simulink model "pfb_fir_generic_test_sim4"  (R2012b)
settings: Solver=VariableStepDiscrete  StartTime=0.0  StopTime=10.0  RelTol=1e-3
model workspace (MAT data in the model file):
  synci = [0 1 2 3 4 5 6 7 8 9 10 11 ... (589826 elements, 294913x2)]
  din0 = [0 1 2 3 4 5 6 7 8 9 10 11 ... (73730 elements, 36865x2)]
  din1 = [0 1 2 3 4 5 6 7 8 9 10 11 ... (73730 elements, 36865x2)]
  din2 = [0 1 2 3 4 5 6 7 8 9 10 11 ... (73730 elements, 36865x2)]
  din3 = [0 1 2 3 4 5 6 7 8 9 10 11 ... (73730 elements, 36865x2)]
  din4 = [0 1 2 3 4 5 6 7 8 9 10 11 ... (73730 elements, 36865x2)]
  din5 = [0 1 2 3 4 5 6 7 8 9 10 11 ... (73730 elements, 36865x2)]
  din6 = [0 1 2 3 4 5 6 7 8 9 10 11 ... (73730 elements, 36865x2)]
  din7 = [0 1 2 3 4 5 6 7 8 9 10 11 ... (73730 elements, 36865x2)]
libraries: xbsIndex_r4 x5323, casper_library_delays x1
(part 16 of 23)

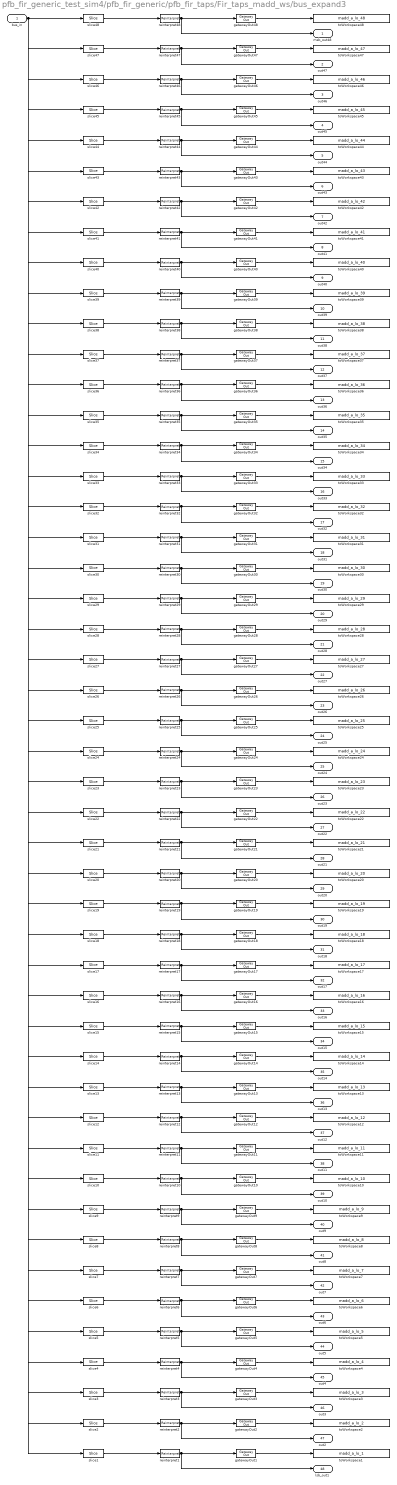
== system pfb_fir_generic_test_sim4/pfb_fir_generic/pfb_fir_taps/Fir_taps_madd_ws/bus_expand3 ==
  bus_in : Inport
  gatewayOut{1..48} (48 alike) : xbsIndex_r4/Gateway Out  inherit_from_input=off  hdl_port=off  timing_constraint=None  locs_specified=off  LOCs={}  UseAsDAC=off  DACChannel='1'  block_type=gatewayout
  reinterpret{1..48} (48 alike) : xbsIndex_r4/Reinterpret  force_arith_type=on  arith_type="Signed  (2's comp)"  force_bin_pt=on  bin_pt=9  block_type=reinterpret
  slice1 : xbsIndex_r4/Slice  nbits=10  boolean_output=off  mode=Upper Bit Location + Width  bit1=-470  base1=MSB of Input  bit0=0  base0=LSB of Input  dbl_ovrd=off  block_type=slice
  slice10 : xbsIndex_r4/Slice  nbits=10  boolean_output=off  mode=Upper Bit Location + Width  bit1=-380  base1=MSB of Input  bit0=0  base0=LSB of Input  dbl_ovrd=off  block_type=slice
  slice11 : xbsIndex_r4/Slice  nbits=10  boolean_output=off  mode=Upper Bit Location + Width  bit1=-370  base1=MSB of Input  bit0=0  base0=LSB of Input  dbl_ovrd=off  block_type=slice
  slice12 : xbsIndex_r4/Slice  nbits=10  boolean_output=off  mode=Upper Bit Location + Width  bit1=-360  base1=MSB of Input  bit0=0  base0=LSB of Input  dbl_ovrd=off  block_type=slice
  slice13 : xbsIndex_r4/Slice  nbits=10  boolean_output=off  mode=Upper Bit Location + Width  bit1=-350  base1=MSB of Input  bit0=0  base0=LSB of Input  dbl_ovrd=off  block_type=slice
  slice14 : xbsIndex_r4/Slice  nbits=10  boolean_output=off  mode=Upper Bit Location + Width  bit1=-340  base1=MSB of Input  bit0=0  base0=LSB of Input  dbl_ovrd=off  block_type=slice
  slice15 : xbsIndex_r4/Slice  nbits=10  boolean_output=off  mode=Upper Bit Location + Width  bit1=-330  base1=MSB of Input  bit0=0  base0=LSB of Input  dbl_ovrd=off  block_type=slice
  slice16 : xbsIndex_r4/Slice  nbits=10  boolean_output=off  mode=Upper Bit Location + Width  bit1=-320  base1=MSB of Input  bit0=0  base0=LSB of Input  dbl_ovrd=off  block_type=slice
  slice17 : xbsIndex_r4/Slice  nbits=10  boolean_output=off  mode=Upper Bit Location + Width  bit1=-310  base1=MSB of Input  bit0=0  base0=LSB of Input  dbl_ovrd=off  block_type=slice
  slice18 : xbsIndex_r4/Slice  nbits=10  boolean_output=off  mode=Upper Bit Location + Width  bit1=-300  base1=MSB of Input  bit0=0  base0=LSB of Input  dbl_ovrd=off  block_type=slice
  slice19 : xbsIndex_r4/Slice  nbits=10  boolean_output=off  mode=Upper Bit Location + Width  bit1=-290  base1=MSB of Input  bit0=0  base0=LSB of Input  dbl_ovrd=off  block_type=slice
  slice2 : xbsIndex_r4/Slice  nbits=10  boolean_output=off  mode=Upper Bit Location + Width  bit1=-460  base1=MSB of Input  bit0=0  base0=LSB of Input  dbl_ovrd=off  block_type=slice
  slice20 : xbsIndex_r4/Slice  nbits=10  boolean_output=off  mode=Upper Bit Location + Width  bit1=-280  base1=MSB of Input  bit0=0  base0=LSB of Input  dbl_ovrd=off  block_type=slice
  slice21 : xbsIndex_r4/Slice  nbits=10  boolean_output=off  mode=Upper Bit Location + Width  bit1=-270  base1=MSB of Input  bit0=0  base0=LSB of Input  dbl_ovrd=off  block_type=slice
  slice22 : xbsIndex_r4/Slice  nbits=10  boolean_output=off  mode=Upper Bit Location + Width  bit1=-260  base1=MSB of Input  bit0=0  base0=LSB of Input  dbl_ovrd=off  block_type=slice
  slice23 : xbsIndex_r4/Slice  nbits=10  boolean_output=off  mode=Upper Bit Location + Width  bit1=-250  base1=MSB of Input  bit0=0  base0=LSB of Input  dbl_ovrd=off  block_type=slice
  slice24 : xbsIndex_r4/Slice  nbits=10  boolean_output=off  mode=Upper Bit Location + Width  bit1=-240  base1=MSB of Input  bit0=0  base0=LSB of Input  dbl_ovrd=off  block_type=slice
  slice25 : xbsIndex_r4/Slice  nbits=10  boolean_output=off  mode=Upper Bit Location + Width  bit1=-230  base1=MSB of Input  bit0=0  base0=LSB of Input  dbl_ovrd=off  block_type=slice
  slice26 : xbsIndex_r4/Slice  nbits=10  boolean_output=off  mode=Upper Bit Location + Width  bit1=-220  base1=MSB of Input  bit0=0  base0=LSB of Input  dbl_ovrd=off  block_type=slice
  slice27 : xbsIndex_r4/Slice  nbits=10  boolean_output=off  mode=Upper Bit Location + Width  bit1=-210  base1=MSB of Input  bit0=0  base0=LSB of Input  dbl_ovrd=off  block_type=slice
  slice28 : xbsIndex_r4/Slice  nbits=10  boolean_output=off  mode=Upper Bit Location + Width  bit1=-200  base1=MSB of Input  bit0=0  base0=LSB of Input  dbl_ovrd=off  block_type=slice
  slice29 : xbsIndex_r4/Slice  nbits=10  boolean_output=off  mode=Upper Bit Location + Width  bit1=-190  base1=MSB of Input  bit0=0  base0=LSB of Input  dbl_ovrd=off  block_type=slice
  slice3 : xbsIndex_r4/Slice  nbits=10  boolean_output=off  mode=Upper Bit Location + Width  bit1=-450  base1=MSB of Input  bit0=0  base0=LSB of Input  dbl_ovrd=off  block_type=slice
  slice30 : xbsIndex_r4/Slice  nbits=10  boolean_output=off  mode=Upper Bit Location + Width  bit1=-180  base1=MSB of Input  bit0=0  base0=LSB of Input  dbl_ovrd=off  block_type=slice
  slice31 : xbsIndex_r4/Slice  nbits=10  boolean_output=off  mode=Upper Bit Location + Width  bit1=-170  base1=MSB of Input  bit0=0  base0=LSB of Input  dbl_ovrd=off  block_type=slice
  slice32 : xbsIndex_r4/Slice  nbits=10  boolean_output=off  mode=Upper Bit Location + Width  bit1=-160  base1=MSB of Input  bit0=0  base0=LSB of Input  dbl_ovrd=off  block_type=slice
  slice33 : xbsIndex_r4/Slice  nbits=10  boolean_output=off  mode=Upper Bit Location + Width  bit1=-150  base1=MSB of Input  bit0=0  base0=LSB of Input  dbl_ovrd=off  block_type=slice
  slice34 : xbsIndex_r4/Slice  nbits=10  boolean_output=off  mode=Upper Bit Location + Width  bit1=-140  base1=MSB of Input  bit0=0  base0=LSB of Input  dbl_ovrd=off  block_type=slice
  slice35 : xbsIndex_r4/Slice  nbits=10  boolean_output=off  mode=Upper Bit Location + Width  bit1=-130  base1=MSB of Input  bit0=0  base0=LSB of Input  dbl_ovrd=off  block_type=slice
  slice36 : xbsIndex_r4/Slice  nbits=10  boolean_output=off  mode=Upper Bit Location + Width  bit1=-120  base1=MSB of Input  bit0=0  base0=LSB of Input  dbl_ovrd=off  block_type=slice
  slice37 : xbsIndex_r4/Slice  nbits=10  boolean_output=off  mode=Upper Bit Location + Width  bit1=-110  base1=MSB of Input  bit0=0  base0=LSB of Input  dbl_ovrd=off  block_type=slice
  slice38 : xbsIndex_r4/Slice  nbits=10  boolean_output=off  mode=Upper Bit Location + Width  bit1=-100  base1=MSB of Input  bit0=0  base0=LSB of Input  dbl_ovrd=off  block_type=slice
  slice39 : xbsIndex_r4/Slice  nbits=10  boolean_output=off  mode=Upper Bit Location + Width  bit1=-90  base1=MSB of Input  bit0=0  base0=LSB of Input  dbl_ovrd=off  block_type=slice
  slice4 : xbsIndex_r4/Slice  nbits=10  boolean_output=off  mode=Upper Bit Location + Width  bit1=-440  base1=MSB of Input  bit0=0  base0=LSB of Input  dbl_ovrd=off  block_type=slice
  slice40 : xbsIndex_r4/Slice  nbits=10  boolean_output=off  mode=Upper Bit Location + Width  bit1=-80  base1=MSB of Input  bit0=0  base0=LSB of Input  dbl_ovrd=off  block_type=slice
  slice41 : xbsIndex_r4/Slice  nbits=10  boolean_output=off  mode=Upper Bit Location + Width  bit1=-70  base1=MSB of Input  bit0=0  base0=LSB of Input  dbl_ovrd=off  block_type=slice
  slice42 : xbsIndex_r4/Slice  nbits=10  boolean_output=off  mode=Upper Bit Location + Width  bit1=-60  base1=MSB of Input  bit0=0  base0=LSB of Input  dbl_ovrd=off  block_type=slice
  slice43 : xbsIndex_r4/Slice  nbits=10  boolean_output=off  mode=Upper Bit Location + Width  bit1=-50  base1=MSB of Input  bit0=0  base0=LSB of Input  dbl_ovrd=off  block_type=slice
  slice44 : xbsIndex_r4/Slice  nbits=10  boolean_output=off  mode=Upper Bit Location + Width  bit1=-40  base1=MSB of Input  bit0=0  base0=LSB of Input  dbl_ovrd=off  block_type=slice
  slice45 : xbsIndex_r4/Slice  nbits=10  boolean_output=off  mode=Upper Bit Location + Width  bit1=-30  base1=MSB of Input  bit0=0  base0=LSB of Input  dbl_ovrd=off  block_type=slice
  slice46 : xbsIndex_r4/Slice  nbits=10  boolean_output=off  mode=Upper Bit Location + Width  bit1=-20  base1=MSB of Input  bit0=0  base0=LSB of Input  dbl_ovrd=off  block_type=slice
  slice47 : xbsIndex_r4/Slice  nbits=10  boolean_output=off  mode=Upper Bit Location + Width  bit1=-10  base1=MSB of Input  bit0=0  base0=LSB of Input  dbl_ovrd=off  block_type=slice
  slice48 : xbsIndex_r4/Slice  nbits=10  boolean_output=off  mode=Upper Bit Location + Width  bit1=0  base1=MSB of Input  bit0=0  base0=LSB of Input  dbl_ovrd=off  block_type=slice
  slice5 : xbsIndex_r4/Slice  nbits=10  boolean_output=off  mode=Upper Bit Location + Width  bit1=-430  base1=MSB of Input  bit0=0  base0=LSB of Input  dbl_ovrd=off  block_type=slice
  slice6 : xbsIndex_r4/Slice  nbits=10  boolean_output=off  mode=Upper Bit Location + Width  bit1=-420  base1=MSB of Input  bit0=0  base0=LSB of Input  dbl_ovrd=off  block_type=slice
  slice7 : xbsIndex_r4/Slice  nbits=10  boolean_output=off  mode=Upper Bit Location + Width  bit1=-410  base1=MSB of Input  bit0=0  base0=LSB of Input  dbl_ovrd=off  block_type=slice
  slice8 : xbsIndex_r4/Slice  nbits=10  boolean_output=off  mode=Upper Bit Location + Width  bit1=-400  base1=MSB of Input  bit0=0  base0=LSB of Input  dbl_ovrd=off  block_type=slice
  slice9 : xbsIndex_r4/Slice  nbits=10  boolean_output=off  mode=Upper Bit Location + Width  bit1=-390  base1=MSB of Input  bit0=0  base0=LSB of Input  dbl_ovrd=off  block_type=slice
  toWorkspace1 : ToWorkspace  VariableName=madd_a_lo_1  SampleTime=-1  SaveFormat=Structure With Time
  toWorkspace10 : ToWorkspace  VariableName=madd_a_lo_10  SampleTime=-1  SaveFormat=Structure With Time
  toWorkspace11 : ToWorkspace  VariableName=madd_a_lo_11  SampleTime=-1  SaveFormat=Structure With Time
  toWorkspace12 : ToWorkspace  VariableName=madd_a_lo_12  SampleTime=-1  SaveFormat=Structure With Time
  toWorkspace13 : ToWorkspace  VariableName=madd_a_lo_13  SampleTime=-1  SaveFormat=Structure With Time
  toWorkspace14 : ToWorkspace  VariableName=madd_a_lo_14  SampleTime=-1  SaveFormat=Structure With Time
  toWorkspace15 : ToWorkspace  VariableName=madd_a_lo_15  SampleTime=-1  SaveFormat=Structure With Time
  toWorkspace16 : ToWorkspace  VariableName=madd_a_lo_16  SampleTime=-1  SaveFormat=Structure With Time
  toWorkspace17 : ToWorkspace  VariableName=madd_a_lo_17  SampleTime=-1  SaveFormat=Structure With Time
  toWorkspace18 : ToWorkspace  VariableName=madd_a_lo_18  SampleTime=-1  SaveFormat=Structure With Time
  toWorkspace19 : ToWorkspace  VariableName=madd_a_lo_19  SampleTime=-1  SaveFormat=Structure With Time
  toWorkspace2 : ToWorkspace  VariableName=madd_a_lo_2  SampleTime=-1  SaveFormat=Structure With Time
  toWorkspace20 : ToWorkspace  VariableName=madd_a_lo_20  SampleTime=-1  SaveFormat=Structure With Time
  toWorkspace21 : ToWorkspace  VariableName=madd_a_lo_21  SampleTime=-1  SaveFormat=Structure With Time
  toWorkspace22 : ToWorkspace  VariableName=madd_a_lo_22  SampleTime=-1  SaveFormat=Structure With Time
  toWorkspace23 : ToWorkspace  VariableName=madd_a_lo_23  SampleTime=-1  SaveFormat=Structure With Time
  toWorkspace24 : ToWorkspace  VariableName=madd_a_lo_24  SampleTime=-1  SaveFormat=Structure With Time
  toWorkspace25 : ToWorkspace  VariableName=madd_a_lo_25  SampleTime=-1  SaveFormat=Structure With Time
  toWorkspace26 : ToWorkspace  VariableName=madd_a_lo_26  SampleTime=-1  SaveFormat=Structure With Time
  toWorkspace27 : ToWorkspace  VariableName=madd_a_lo_27  SampleTime=-1  SaveFormat=Structure With Time
  toWorkspace28 : ToWorkspace  VariableName=madd_a_lo_28  SampleTime=-1  SaveFormat=Structure With Time
  toWorkspace29 : ToWorkspace  VariableName=madd_a_lo_29  SampleTime=-1  SaveFormat=Structure With Time
  toWorkspace3 : ToWorkspace  VariableName=madd_a_lo_3  SampleTime=-1  SaveFormat=Structure With Time
  toWorkspace30 : ToWorkspace  VariableName=madd_a_lo_30  SampleTime=-1  SaveFormat=Structure With Time
  toWorkspace31 : ToWorkspace  VariableName=madd_a_lo_31  SampleTime=-1  SaveFormat=Structure With Time
  toWorkspace32 : ToWorkspace  VariableName=madd_a_lo_32  SampleTime=-1  SaveFormat=Structure With Time
  toWorkspace33 : ToWorkspace  VariableName=madd_a_lo_33  SampleTime=-1  SaveFormat=Structure With Time
  toWorkspace34 : ToWorkspace  VariableName=madd_a_lo_34  SampleTime=-1  SaveFormat=Structure With Time
  toWorkspace35 : ToWorkspace  VariableName=madd_a_lo_35  SampleTime=-1  SaveFormat=Structure With Time
  toWorkspace36 : ToWorkspace  VariableName=madd_a_lo_36  SampleTime=-1  SaveFormat=Structure With Time
  toWorkspace37 : ToWorkspace  VariableName=madd_a_lo_37  SampleTime=-1  SaveFormat=Structure With Time
  toWorkspace38 : ToWorkspace  VariableName=madd_a_lo_38  SampleTime=-1  SaveFormat=Structure With Time
  toWorkspace39 : ToWorkspace  VariableName=madd_a_lo_39  SampleTime=-1  SaveFormat=Structure With Time
  toWorkspace4 : ToWorkspace  VariableName=madd_a_lo_4  SampleTime=-1  SaveFormat=Structure With Time
  toWorkspace40 : ToWorkspace  VariableName=madd_a_lo_40  SampleTime=-1  SaveFormat=Structure With Time
  toWorkspace41 : ToWorkspace  VariableName=madd_a_lo_41  SampleTime=-1  SaveFormat=Structure With Time
  toWorkspace42 : ToWorkspace  VariableName=madd_a_lo_42  SampleTime=-1  SaveFormat=Structure With Time
  toWorkspace43 : ToWorkspace  VariableName=madd_a_lo_43  SampleTime=-1  SaveFormat=Structure With Time
  toWorkspace44 : ToWorkspace  VariableName=madd_a_lo_44  SampleTime=-1  SaveFormat=Structure With Time
  toWorkspace45 : ToWorkspace  VariableName=madd_a_lo_45  SampleTime=-1  SaveFormat=Structure With Time
  toWorkspace46 : ToWorkspace  VariableName=madd_a_lo_46  SampleTime=-1  SaveFormat=Structure With Time
  toWorkspace47 : ToWorkspace  VariableName=madd_a_lo_47  SampleTime=-1  SaveFormat=Structure With Time
  toWorkspace48 : ToWorkspace  VariableName=madd_a_lo_48  SampleTime=-1  SaveFormat=Structure With Time
  toWorkspace5 : ToWorkspace  VariableName=madd_a_lo_5  SampleTime=-1  SaveFormat=Structure With Time
  toWorkspace6 : ToWorkspace  VariableName=madd_a_lo_6  SampleTime=-1  SaveFormat=Structure With Time
  toWorkspace7 : ToWorkspace  VariableName=madd_a_lo_7  SampleTime=-1  SaveFormat=Structure With Time
  toWorkspace8 : ToWorkspace  VariableName=madd_a_lo_8  SampleTime=-1  SaveFormat=Structure With Time
  toWorkspace9 : ToWorkspace  VariableName=madd_a_lo_9  SampleTime=-1  SaveFormat=Structure With Time
  msb_out48 : Outport
  out47 : Outport  Port=2
  out46 : Outport  Port=3
  out45 : Outport  Port=4
  out44 : Outport  Port=5
  out43 : Outport  Port=6
  out42 : Outport  Port=7
  out41 : Outport  Port=8
  out40 : Outport  Port=9
  out39 : Outport  Port=10
  out38 : Outport  Port=11
  out37 : Outport  Port=12
  out36 : Outport  Port=13
  out35 : Outport  Port=14
  out34 : Outport  Port=15
  out33 : Outport  Port=16
  out32 : Outport  Port=17
  out31 : Outport  Port=18
  out30 : Outport  Port=19
  out29 : Outport  Port=20
  out28 : Outport  Port=21
  out27 : Outport  Port=22
  out26 : Outport  Port=23
  out25 : Outport  Port=24
  out24 : Outport  Port=25
  out23 : Outport  Port=26
  out22 : Outport  Port=27
  out21 : Outport  Port=28
  out20 : Outport  Port=29
  out19 : Outport  Port=30
  out18 : Outport  Port=31
  out17 : Outport  Port=32
  out16 : Outport  Port=33
  out15 : Outport  Port=34
  out14 : Outport  Port=35
  out13 : Outport  Port=36
  out12 : Outport  Port=37
  out11 : Outport  Port=38
  out10 : Outport  Port=39
  out9 : Outport  Port=40
  out8 : Outport  Port=41
  out7 : Outport  Port=42
  out6 : Outport  Port=43
  out5 : Outport  Port=44
  out4 : Outport  Port=45
  out3 : Outport  Port=46
  out2 : Outport  Port=47
  lsb_out1 : Outport  Port=48
  wires:
  bus_in/1 -> slice48/1, slice47/1, slice46/1, slice45/1, slice44/1, slice43/1, slice42/1, slice41/1, slice40/1, slice39/1, slice38/1, slice37/1, slice36/1, slice35/1, slice34/1, slice33/1, slice32/1, slice31/1, slice30/1, slice29/1, slice28/1, slice27/1, slice26/1, slice25/1, slice24/1, slice23/1, slice22/1, slice21/1, slice20/1, slice19/1, slice18/1, slice17/1, slice16/1, slice15/1, slice14/1, slice13/1, slice12/1, slice11/1, slice10/1, slice9/1, slice8/1, slice7/1, slice6/1, slice5/1, slice4/1, slice3/1, slice2/1, slice1/1
  slice48/1 -> reinterpret48/1
  reinterpret48/1 -> gatewayOut48/1, msb_out48/1
  gatewayOut48/1 -> toWorkspace48/1
  slice47/1 -> reinterpret47/1
  reinterpret47/1 -> gatewayOut47/1, out47/1
  gatewayOut47/1 -> toWorkspace47/1
  slice46/1 -> reinterpret46/1
  reinterpret46/1 -> gatewayOut46/1, out46/1
  gatewayOut46/1 -> toWorkspace46/1
  slice45/1 -> reinterpret45/1
  reinterpret45/1 -> gatewayOut45/1, out45/1
  gatewayOut45/1 -> toWorkspace45/1
  slice44/1 -> reinterpret44/1
  reinterpret44/1 -> gatewayOut44/1, out44/1
  gatewayOut44/1 -> toWorkspace44/1
  slice43/1 -> reinterpret43/1
  reinterpret43/1 -> gatewayOut43/1, out43/1
  gatewayOut43/1 -> toWorkspace43/1
  slice42/1 -> reinterpret42/1
  reinterpret42/1 -> gatewayOut42/1, out42/1
  gatewayOut42/1 -> toWorkspace42/1
  slice41/1 -> reinterpret41/1
  reinterpret41/1 -> gatewayOut41/1, out41/1
  gatewayOut41/1 -> toWorkspace41/1
  slice40/1 -> reinterpret40/1
  reinterpret40/1 -> gatewayOut40/1, out40/1
  gatewayOut40/1 -> toWorkspace40/1
  slice39/1 -> reinterpret39/1
  reinterpret39/1 -> gatewayOut39/1, out39/1
  gatewayOut39/1 -> toWorkspace39/1
  slice38/1 -> reinterpret38/1
  reinterpret38/1 -> gatewayOut38/1, out38/1
  gatewayOut38/1 -> toWorkspace38/1
  slice37/1 -> reinterpret37/1
  reinterpret37/1 -> gatewayOut37/1, out37/1
  gatewayOut37/1 -> toWorkspace37/1
  slice36/1 -> reinterpret36/1
  reinterpret36/1 -> gatewayOut36/1, out36/1
  gatewayOut36/1 -> toWorkspace36/1
  slice35/1 -> reinterpret35/1
  reinterpret35/1 -> gatewayOut35/1, out35/1
  gatewayOut35/1 -> toWorkspace35/1
  slice34/1 -> reinterpret34/1
  reinterpret34/1 -> gatewayOut34/1, out34/1
  gatewayOut34/1 -> toWorkspace34/1
  slice33/1 -> reinterpret33/1
  reinterpret33/1 -> gatewayOut33/1, out33/1
  gatewayOut33/1 -> toWorkspace33/1
  slice32/1 -> reinterpret32/1
  reinterpret32/1 -> gatewayOut32/1, out32/1
  gatewayOut32/1 -> toWorkspace32/1
  slice31/1 -> reinterpret31/1
  reinterpret31/1 -> gatewayOut31/1, out31/1
  gatewayOut31/1 -> toWorkspace31/1
  slice30/1 -> reinterpret30/1
  reinterpret30/1 -> gatewayOut30/1, out30/1
  gatewayOut30/1 -> toWorkspace30/1
  slice29/1 -> reinterpret29/1
  reinterpret29/1 -> gatewayOut29/1, out29/1
  gatewayOut29/1 -> toWorkspace29/1
  slice28/1 -> reinterpret28/1
  reinterpret28/1 -> gatewayOut28/1, out28/1
  gatewayOut28/1 -> toWorkspace28/1
  slice27/1 -> reinterpret27/1
  reinterpret27/1 -> gatewayOut27/1, out27/1
  gatewayOut27/1 -> toWorkspace27/1
  slice26/1 -> reinterpret26/1
  reinterpret26/1 -> gatewayOut26/1, out26/1
  gatewayOut26/1 -> toWorkspace26/1
  slice25/1 -> reinterpret25/1
  reinterpret25/1 -> gatewayOut25/1, out25/1
  gatewayOut25/1 -> toWorkspace25/1
  slice24/1 -> reinterpret24/1
  reinterpret24/1 -> gatewayOut24/1, out24/1
  gatewayOut24/1 -> toWorkspace24/1
  slice23/1 -> reinterpret23/1
  reinterpret23/1 -> gatewayOut23/1, out23/1
  gatewayOut23/1 -> toWorkspace23/1
  slice22/1 -> reinterpret22/1
  reinterpret22/1 -> gatewayOut22/1, out22/1
  gatewayOut22/1 -> toWorkspace22/1
  slice21/1 -> reinterpret21/1
  reinterpret21/1 -> gatewayOut21/1, out21/1
  gatewayOut21/1 -> toWorkspace21/1
  slice20/1 -> reinterpret20/1
  reinterpret20/1 -> gatewayOut20/1, out20/1
  gatewayOut20/1 -> toWorkspace20/1
  slice19/1 -> reinterpret19/1
  reinterpret19/1 -> gatewayOut19/1, out19/1
  gatewayOut19/1 -> toWorkspace19/1
  slice18/1 -> reinterpret18/1
  reinterpret18/1 -> gatewayOut18/1, out18/1
  gatewayOut18/1 -> toWorkspace18/1
  slice17/1 -> reinterpret17/1
  reinterpret17/1 -> gatewayOut17/1, out17/1
  gatewayOut17/1 -> toWorkspace17/1
  slice16/1 -> reinterpret16/1
  reinterpret16/1 -> gatewayOut16/1, out16/1
  gatewayOut16/1 -> toWorkspace16/1
  slice15/1 -> reinterpret15/1
  reinterpret15/1 -> gatewayOut15/1, out15/1
  gatewayOut15/1 -> toWorkspace15/1
  slice14/1 -> reinterpret14/1
  reinterpret14/1 -> gatewayOut14/1, out14/1
  gatewayOut14/1 -> toWorkspace14/1
  slice13/1 -> reinterpret13/1
  reinterpret13/1 -> gatewayOut13/1, out13/1
  gatewayOut13/1 -> toWorkspace13/1
  slice12/1 -> reinterpret12/1
  reinterpret12/1 -> gatewayOut12/1, out12/1
  gatewayOut12/1 -> toWorkspace12/1
  slice11/1 -> reinterpret11/1
  reinterpret11/1 -> gatewayOut11/1, out11/1
  gatewayOut11/1 -> toWorkspace11/1
  slice10/1 -> reinterpret10/1
  reinterpret10/1 -> gatewayOut10/1, out10/1
  gatewayOut10/1 -> toWorkspace10/1
  slice9/1 -> reinterpret9/1
  reinterpret9/1 -> gatewayOut9/1, out9/1
  gatewayOut9/1 -> toWorkspace9/1
  slice8/1 -> reinterpret8/1
  reinterpret8/1 -> gatewayOut8/1, out8/1
  gatewayOut8/1 -> toWorkspace8/1
  slice7/1 -> reinterpret7/1
  reinterpret7/1 -> gatewayOut7/1, out7/1
  gatewayOut7/1 -> toWorkspace7/1
  slice6/1 -> reinterpret6/1
  reinterpret6/1 -> gatewayOut6/1, out6/1
  gatewayOut6/1 -> toWorkspace6/1
  slice5/1 -> reinterpret5/1
  reinterpret5/1 -> gatewayOut5/1, out5/1
  gatewayOut5/1 -> toWorkspace5/1
  slice4/1 -> reinterpret4/1
  reinterpret4/1 -> gatewayOut4/1, out4/1
  gatewayOut4/1 -> toWorkspace4/1
  slice3/1 -> reinterpret3/1
  reinterpret3/1 -> gatewayOut3/1, out3/1
  gatewayOut3/1 -> toWorkspace3/1
  slice2/1 -> reinterpret2/1
  reinterpret2/1 -> gatewayOut2/1, out2/1
  gatewayOut2/1 -> toWorkspace2/1
  slice1/1 -> reinterpret1/1
  reinterpret1/1 -> gatewayOut1/1, lsb_out1/1
  gatewayOut1/1 -> toWorkspace1/1

== system pfb_fir_generic_test_sim4/pfb_fir_generic/pfb_fir_taps/Fir_taps_madd_ws/bus_expand4 ==
  bus_in : Inport
  gatewayOut{1..16} (16 alike) : xbsIndex_r4/Gateway Out  inherit_from_input=off  hdl_port=off  timing_constraint=None  locs_specified=off  LOCs={}  UseAsDAC=off  DACChannel='1'  block_type=gatewayout
  reinterpret{1..16} (16 alike) : xbsIndex_r4/Reinterpret  force_arith_type=on  arith_type="Signed  (2's comp)"  force_bin_pt=on  bin_pt=9  block_type=reinterpret
  slice1 : xbsIndex_r4/Slice  nbits=10  boolean_output=off  mode=Upper Bit Location + Width  bit1=-150  base1=MSB of Input  bit0=0  base0=LSB of Input  dbl_ovrd=off  block_type=slice
  slice10 : xbsIndex_r4/Slice  nbits=10  boolean_output=off  mode=Upper Bit Location + Width  bit1=-60  base1=MSB of Input  bit0=0  base0=LSB of Input  dbl_ovrd=off  block_type=slice
  slice11 : xbsIndex_r4/Slice  nbits=10  boolean_output=off  mode=Upper Bit Location + Width  bit1=-50  base1=MSB of Input  bit0=0  base0=LSB of Input  dbl_ovrd=off  block_type=slice
  slice12 : xbsIndex_r4/Slice  nbits=10  boolean_output=off  mode=Upper Bit Location + Width  bit1=-40  base1=MSB of Input  bit0=0  base0=LSB of Input  dbl_ovrd=off  block_type=slice
  slice13 : xbsIndex_r4/Slice  nbits=10  boolean_output=off  mode=Upper Bit Location + Width  bit1=-30  base1=MSB of Input  bit0=0  base0=LSB of Input  dbl_ovrd=off  block_type=slice
  slice14 : xbsIndex_r4/Slice  nbits=10  boolean_output=off  mode=Upper Bit Location + Width  bit1=-20  base1=MSB of Input  bit0=0  base0=LSB of Input  dbl_ovrd=off  block_type=slice
  slice15 : xbsIndex_r4/Slice  nbits=10  boolean_output=off  mode=Upper Bit Location + Width  bit1=-10  base1=MSB of Input  bit0=0  base0=LSB of Input  dbl_ovrd=off  block_type=slice
  slice16 : xbsIndex_r4/Slice  nbits=10  boolean_output=off  mode=Upper Bit Location + Width  bit1=0  base1=MSB of Input  bit0=0  base0=LSB of Input  dbl_ovrd=off  block_type=slice
  slice2 : xbsIndex_r4/Slice  nbits=10  boolean_output=off  mode=Upper Bit Location + Width  bit1=-140  base1=MSB of Input  bit0=0  base0=LSB of Input  dbl_ovrd=off  block_type=slice
  slice3 : xbsIndex_r4/Slice  nbits=10  boolean_output=off  mode=Upper Bit Location + Width  bit1=-130  base1=MSB of Input  bit0=0  base0=LSB of Input  dbl_ovrd=off  block_type=slice
  slice4 : xbsIndex_r4/Slice  nbits=10  boolean_output=off  mode=Upper Bit Location + Width  bit1=-120  base1=MSB of Input  bit0=0  base0=LSB of Input  dbl_ovrd=off  block_type=slice
  slice5 : xbsIndex_r4/Slice  nbits=10  boolean_output=off  mode=Upper Bit Location + Width  bit1=-110  base1=MSB of Input  bit0=0  base0=LSB of Input  dbl_ovrd=off  block_type=slice
  slice6 : xbsIndex_r4/Slice  nbits=10  boolean_output=off  mode=Upper Bit Location + Width  bit1=-100  base1=MSB of Input  bit0=0  base0=LSB of Input  dbl_ovrd=off  block_type=slice
  slice7 : xbsIndex_r4/Slice  nbits=10  boolean_output=off  mode=Upper Bit Location + Width  bit1=-90  base1=MSB of Input  bit0=0  base0=LSB of Input  dbl_ovrd=off  block_type=slice
  slice8 : xbsIndex_r4/Slice  nbits=10  boolean_output=off  mode=Upper Bit Location + Width  bit1=-80  base1=MSB of Input  bit0=0  base0=LSB of Input  dbl_ovrd=off  block_type=slice
  slice9 : xbsIndex_r4/Slice  nbits=10  boolean_output=off  mode=Upper Bit Location + Width  bit1=-70  base1=MSB of Input  bit0=0  base0=LSB of Input  dbl_ovrd=off  block_type=slice
  toWorkspace1 : ToWorkspace  VariableName=delay_bram_din_hi_1  SampleTime=-1  SaveFormat=Structure With Time
  toWorkspace10 : ToWorkspace  VariableName=delay_bram_din_hi_10  SampleTime=-1  SaveFormat=Structure With Time
  toWorkspace11 : ToWorkspace  VariableName=delay_bram_din_hi_11  SampleTime=-1  SaveFormat=Structure With Time
  toWorkspace12 : ToWorkspace  VariableName=delay_bram_din_hi_12  SampleTime=-1  SaveFormat=Structure With Time
  toWorkspace13 : ToWorkspace  VariableName=delay_bram_din_hi_13  SampleTime=-1  SaveFormat=Structure With Time
  toWorkspace14 : ToWorkspace  VariableName=delay_bram_din_hi_14  SampleTime=-1  SaveFormat=Structure With Time
  toWorkspace15 : ToWorkspace  VariableName=delay_bram_din_hi_15  SampleTime=-1  SaveFormat=Structure With Time
  toWorkspace16 : ToWorkspace  VariableName=delay_bram_din_hi_16  SampleTime=-1  SaveFormat=Structure With Time
  toWorkspace2 : ToWorkspace  VariableName=delay_bram_din_hi_2  SampleTime=-1  SaveFormat=Structure With Time
  toWorkspace3 : ToWorkspace  VariableName=delay_bram_din_hi_3  SampleTime=-1  SaveFormat=Structure With Time
  toWorkspace4 : ToWorkspace  VariableName=delay_bram_din_hi_4  SampleTime=-1  SaveFormat=Structure With Time
  toWorkspace5 : ToWorkspace  VariableName=delay_bram_din_hi_5  SampleTime=-1  SaveFormat=Structure With Time
  toWorkspace6 : ToWorkspace  VariableName=delay_bram_din_hi_6  SampleTime=-1  SaveFormat=Structure With Time
  toWorkspace7 : ToWorkspace  VariableName=delay_bram_din_hi_7  SampleTime=-1  SaveFormat=Structure With Time
  toWorkspace8 : ToWorkspace  VariableName=delay_bram_din_hi_8  SampleTime=-1  SaveFormat=Structure With Time
  toWorkspace9 : ToWorkspace  VariableName=delay_bram_din_hi_9  SampleTime=-1  SaveFormat=Structure With Time
  msb_out16 : Outport
  out15 : Outport  Port=2
  out14 : Outport  Port=3
  out13 : Outport  Port=4
  out12 : Outport  Port=5
  out11 : Outport  Port=6
  out10 : Outport  Port=7
  out9 : Outport  Port=8
  out8 : Outport  Port=9
  out7 : Outport  Port=10
  out6 : Outport  Port=11
  out5 : Outport  Port=12
  out4 : Outport  Port=13
  out3 : Outport  Port=14
  out2 : Outport  Port=15
  lsb_out1 : Outport  Port=16
  wires:
  bus_in/1 -> slice16/1, slice15/1, slice14/1, slice13/1, slice12/1, slice11/1, slice10/1, slice9/1, slice8/1, slice7/1, slice6/1, slice5/1, slice4/1, slice3/1, slice2/1, slice1/1
  slice16/1 -> reinterpret16/1
  reinterpret16/1 -> gatewayOut16/1, msb_out16/1
  gatewayOut16/1 -> toWorkspace16/1
  slice15/1 -> reinterpret15/1
  reinterpret15/1 -> gatewayOut15/1, out15/1
  gatewayOut15/1 -> toWorkspace15/1
  slice14/1 -> reinterpret14/1
  reinterpret14/1 -> gatewayOut14/1, out14/1
  gatewayOut14/1 -> toWorkspace14/1
  slice13/1 -> reinterpret13/1
  reinterpret13/1 -> gatewayOut13/1, out13/1
  gatewayOut13/1 -> toWorkspace13/1
  slice12/1 -> reinterpret12/1
  reinterpret12/1 -> gatewayOut12/1, out12/1
  gatewayOut12/1 -> toWorkspace12/1
  slice11/1 -> reinterpret11/1
  reinterpret11/1 -> gatewayOut11/1, out11/1
  gatewayOut11/1 -> toWorkspace11/1
  slice10/1 -> reinterpret10/1
  reinterpret10/1 -> gatewayOut10/1, out10/1
  gatewayOut10/1 -> toWorkspace10/1
  slice9/1 -> reinterpret9/1
  reinterpret9/1 -> gatewayOut9/1, out9/1
  gatewayOut9/1 -> toWorkspace9/1
  slice8/1 -> reinterpret8/1
  reinterpret8/1 -> gatewayOut8/1, out8/1
  gatewayOut8/1 -> toWorkspace8/1
  slice7/1 -> reinterpret7/1
  reinterpret7/1 -> gatewayOut7/1, out7/1
  gatewayOut7/1 -> toWorkspace7/1
  slice6/1 -> reinterpret6/1
  reinterpret6/1 -> gatewayOut6/1, out6/1
  gatewayOut6/1 -> toWorkspace6/1
  slice5/1 -> reinterpret5/1
  reinterpret5/1 -> gatewayOut5/1, out5/1
  gatewayOut5/1 -> toWorkspace5/1
  slice4/1 -> reinterpret4/1
  reinterpret4/1 -> gatewayOut4/1, out4/1
  gatewayOut4/1 -> toWorkspace4/1
  slice3/1 -> reinterpret3/1
  reinterpret3/1 -> gatewayOut3/1, out3/1
  gatewayOut3/1 -> toWorkspace3/1
  slice2/1 -> reinterpret2/1
  reinterpret2/1 -> gatewayOut2/1, out2/1
  gatewayOut2/1 -> toWorkspace2/1
  slice1/1 -> reinterpret1/1
  reinterpret1/1 -> gatewayOut1/1, lsb_out1/1
  gatewayOut1/1 -> toWorkspace1/1

== system pfb_fir_generic_test_sim4/pfb_fir_generic/pfb_fir_taps/Fir_taps_madd_ws/bus_expand5 ==
  bus_in : Inport
  gatewayOut{1..32} (32 alike) : xbsIndex_r4/Gateway Out  inherit_from_input=off  hdl_port=off  timing_constraint=None  locs_specified=off  LOCs={}  UseAsDAC=off  DACChannel='1'  block_type=gatewayout
  reinterpret{1..32} (32 alike) : xbsIndex_r4/Reinterpret  force_arith_type=on  arith_type="Signed  (2's comp)"  force_bin_pt=on  bin_pt=9  block_type=reinterpret
  slice1 : xbsIndex_r4/Slice  nbits=10  boolean_output=off  mode=Upper Bit Location + Width  bit1=-310  base1=MSB of Input  bit0=0  base0=LSB of Input  dbl_ovrd=off  block_type=slice
  slice10 : xbsIndex_r4/Slice  nbits=10  boolean_output=off  mode=Upper Bit Location + Width  bit1=-220  base1=MSB of Input  bit0=0  base0=LSB of Input  dbl_ovrd=off  block_type=slice
  slice11 : xbsIndex_r4/Slice  nbits=10  boolean_output=off  mode=Upper Bit Location + Width  bit1=-210  base1=MSB of Input  bit0=0  base0=LSB of Input  dbl_ovrd=off  block_type=slice
  slice12 : xbsIndex_r4/Slice  nbits=10  boolean_output=off  mode=Upper Bit Location + Width  bit1=-200  base1=MSB of Input  bit0=0  base0=LSB of Input  dbl_ovrd=off  block_type=slice
  slice13 : xbsIndex_r4/Slice  nbits=10  boolean_output=off  mode=Upper Bit Location + Width  bit1=-190  base1=MSB of Input  bit0=0  base0=LSB of Input  dbl_ovrd=off  block_type=slice
  slice14 : xbsIndex_r4/Slice  nbits=10  boolean_output=off  mode=Upper Bit Location + Width  bit1=-180  base1=MSB of Input  bit0=0  base0=LSB of Input  dbl_ovrd=off  block_type=slice
  slice15 : xbsIndex_r4/Slice  nbits=10  boolean_output=off  mode=Upper Bit Location + Width  bit1=-170  base1=MSB of Input  bit0=0  base0=LSB of Input  dbl_ovrd=off  block_type=slice
  slice16 : xbsIndex_r4/Slice  nbits=10  boolean_output=off  mode=Upper Bit Location + Width  bit1=-160  base1=MSB of Input  bit0=0  base0=LSB of Input  dbl_ovrd=off  block_type=slice
  slice17 : xbsIndex_r4/Slice  nbits=10  boolean_output=off  mode=Upper Bit Location + Width  bit1=-150  base1=MSB of Input  bit0=0  base0=LSB of Input  dbl_ovrd=off  block_type=slice
  slice18 : xbsIndex_r4/Slice  nbits=10  boolean_output=off  mode=Upper Bit Location + Width  bit1=-140  base1=MSB of Input  bit0=0  base0=LSB of Input  dbl_ovrd=off  block_type=slice
  slice19 : xbsIndex_r4/Slice  nbits=10  boolean_output=off  mode=Upper Bit Location + Width  bit1=-130  base1=MSB of Input  bit0=0  base0=LSB of Input  dbl_ovrd=off  block_type=slice
  slice2 : xbsIndex_r4/Slice  nbits=10  boolean_output=off  mode=Upper Bit Location + Width  bit1=-300  base1=MSB of Input  bit0=0  base0=LSB of Input  dbl_ovrd=off  block_type=slice
  slice20 : xbsIndex_r4/Slice  nbits=10  boolean_output=off  mode=Upper Bit Location + Width  bit1=-120  base1=MSB of Input  bit0=0  base0=LSB of Input  dbl_ovrd=off  block_type=slice
  slice21 : xbsIndex_r4/Slice  nbits=10  boolean_output=off  mode=Upper Bit Location + Width  bit1=-110  base1=MSB of Input  bit0=0  base0=LSB of Input  dbl_ovrd=off  block_type=slice
  slice22 : xbsIndex_r4/Slice  nbits=10  boolean_output=off  mode=Upper Bit Location + Width  bit1=-100  base1=MSB of Input  bit0=0  base0=LSB of Input  dbl_ovrd=off  block_type=slice
  slice23 : xbsIndex_r4/Slice  nbits=10  boolean_output=off  mode=Upper Bit Location + Width  bit1=-90  base1=MSB of Input  bit0=0  base0=LSB of Input  dbl_ovrd=off  block_type=slice
  slice24 : xbsIndex_r4/Slice  nbits=10  boolean_output=off  mode=Upper Bit Location + Width  bit1=-80  base1=MSB of Input  bit0=0  base0=LSB of Input  dbl_ovrd=off  block_type=slice
  slice25 : xbsIndex_r4/Slice  nbits=10  boolean_output=off  mode=Upper Bit Location + Width  bit1=-70  base1=MSB of Input  bit0=0  base0=LSB of Input  dbl_ovrd=off  block_type=slice
  slice26 : xbsIndex_r4/Slice  nbits=10  boolean_output=off  mode=Upper Bit Location + Width  bit1=-60  base1=MSB of Input  bit0=0  base0=LSB of Input  dbl_ovrd=off  block_type=slice
  slice27 : xbsIndex_r4/Slice  nbits=10  boolean_output=off  mode=Upper Bit Location + Width  bit1=-50  base1=MSB of Input  bit0=0  base0=LSB of Input  dbl_ovrd=off  block_type=slice
  slice28 : xbsIndex_r4/Slice  nbits=10  boolean_output=off  mode=Upper Bit Location + Width  bit1=-40  base1=MSB of Input  bit0=0  base0=LSB of Input  dbl_ovrd=off  block_type=slice
  slice29 : xbsIndex_r4/Slice  nbits=10  boolean_output=off  mode=Upper Bit Location + Width  bit1=-30  base1=MSB of Input  bit0=0  base0=LSB of Input  dbl_ovrd=off  block_type=slice
  slice3 : xbsIndex_r4/Slice  nbits=10  boolean_output=off  mode=Upper Bit Location + Width  bit1=-290  base1=MSB of Input  bit0=0  base0=LSB of Input  dbl_ovrd=off  block_type=slice
  slice30 : xbsIndex_r4/Slice  nbits=10  boolean_output=off  mode=Upper Bit Location + Width  bit1=-20  base1=MSB of Input  bit0=0  base0=LSB of Input  dbl_ovrd=off  block_type=slice
  slice31 : xbsIndex_r4/Slice  nbits=10  boolean_output=off  mode=Upper Bit Location + Width  bit1=-10  base1=MSB of Input  bit0=0  base0=LSB of Input  dbl_ovrd=off  block_type=slice
  slice32 : xbsIndex_r4/Slice  nbits=10  boolean_output=off  mode=Upper Bit Location + Width  bit1=0  base1=MSB of Input  bit0=0  base0=LSB of Input  dbl_ovrd=off  block_type=slice
  slice4 : xbsIndex_r4/Slice  nbits=10  boolean_output=off  mode=Upper Bit Location + Width  bit1=-280  base1=MSB of Input  bit0=0  base0=LSB of Input  dbl_ovrd=off  block_type=slice
  slice5 : xbsIndex_r4/Slice  nbits=10  boolean_output=off  mode=Upper Bit Location + Width  bit1=-270  base1=MSB of Input  bit0=0  base0=LSB of Input  dbl_ovrd=off  block_type=slice
  slice6 : xbsIndex_r4/Slice  nbits=10  boolean_output=off  mode=Upper Bit Location + Width  bit1=-260  base1=MSB of Input  bit0=0  base0=LSB of Input  dbl_ovrd=off  block_type=slice
  slice7 : xbsIndex_r4/Slice  nbits=10  boolean_output=off  mode=Upper Bit Location + Width  bit1=-250  base1=MSB of Input  bit0=0  base0=LSB of Input  dbl_ovrd=off  block_type=slice
  slice8 : xbsIndex_r4/Slice  nbits=10  boolean_output=off  mode=Upper Bit Location + Width  bit1=-240  base1=MSB of Input  bit0=0  base0=LSB of Input  dbl_ovrd=off  block_type=slice
  slice9 : xbsIndex_r4/Slice  nbits=10  boolean_output=off  mode=Upper Bit Location + Width  bit1=-230  base1=MSB of Input  bit0=0  base0=LSB of Input  dbl_ovrd=off  block_type=slice
  toWorkspace1 : ToWorkspace  VariableName=delay_bram_din_lo_1  SampleTime=-1  SaveFormat=Structure With Time
  toWorkspace10 : ToWorkspace  VariableName=delay_bram_din_lo_10  SampleTime=-1  SaveFormat=Structure With Time
  toWorkspace11 : ToWorkspace  VariableName=delay_bram_din_lo_11  SampleTime=-1  SaveFormat=Structure With Time
  toWorkspace12 : ToWorkspace  VariableName=delay_bram_din_lo_12  SampleTime=-1  SaveFormat=Structure With Time
  toWorkspace13 : ToWorkspace  VariableName=delay_bram_din_lo_13  SampleTime=-1  SaveFormat=Structure With Time
  toWorkspace14 : ToWorkspace  VariableName=delay_bram_din_lo_14  SampleTime=-1  SaveFormat=Structure With Time
  toWorkspace15 : ToWorkspace  VariableName=delay_bram_din_lo_15  SampleTime=-1  SaveFormat=Structure With Time
  toWorkspace16 : ToWorkspace  VariableName=delay_bram_din_lo_16  SampleTime=-1  SaveFormat=Structure With Time
  toWorkspace17 : ToWorkspace  VariableName=delay_bram_din_lo_17  SampleTime=-1  SaveFormat=Structure With Time
  toWorkspace18 : ToWorkspace  VariableName=delay_bram_din_lo_18  SampleTime=-1  SaveFormat=Structure With Time
  toWorkspace19 : ToWorkspace  VariableName=delay_bram_din_lo_19  SampleTime=-1  SaveFormat=Structure With Time
  toWorkspace2 : ToWorkspace  VariableName=delay_bram_din_lo_2  SampleTime=-1  SaveFormat=Structure With Time
  toWorkspace20 : ToWorkspace  VariableName=delay_bram_din_lo_20  SampleTime=-1  SaveFormat=Structure With Time
  toWorkspace21 : ToWorkspace  VariableName=delay_bram_din_lo_21  SampleTime=-1  SaveFormat=Structure With Time
  toWorkspace22 : ToWorkspace  VariableName=delay_bram_din_lo_22  SampleTime=-1  SaveFormat=Structure With Time
  toWorkspace23 : ToWorkspace  VariableName=delay_bram_din_lo_23  SampleTime=-1  SaveFormat=Structure With Time
  toWorkspace24 : ToWorkspace  VariableName=delay_bram_din_lo_24  SampleTime=-1  SaveFormat=Structure With Time
  toWorkspace25 : ToWorkspace  VariableName=delay_bram_din_lo_25  SampleTime=-1  SaveFormat=Structure With Time
  toWorkspace26 : ToWorkspace  VariableName=delay_bram_din_lo_26  SampleTime=-1  SaveFormat=Structure With Time
  toWorkspace27 : ToWorkspace  VariableName=delay_bram_din_lo_27  SampleTime=-1  SaveFormat=Structure With Time
  toWorkspace28 : ToWorkspace  VariableName=delay_bram_din_lo_28  SampleTime=-1  SaveFormat=Structure With Time
  toWorkspace29 : ToWorkspace  VariableName=delay_bram_din_lo_29  SampleTime=-1  SaveFormat=Structure With Time
  toWorkspace3 : ToWorkspace  VariableName=delay_bram_din_lo_3  SampleTime=-1  SaveFormat=Structure With Time
  toWorkspace30 : ToWorkspace  VariableName=delay_bram_din_lo_30  SampleTime=-1  SaveFormat=Structure With Time
  toWorkspace31 : ToWorkspace  VariableName=delay_bram_din_lo_31  SampleTime=-1  SaveFormat=Structure With Time
  toWorkspace32 : ToWorkspace  VariableName=delay_bram_din_lo_32  SampleTime=-1  SaveFormat=Structure With Time
  toWorkspace4 : ToWorkspace  VariableName=delay_bram_din_lo_4  SampleTime=-1  SaveFormat=Structure With Time
  toWorkspace5 : ToWorkspace  VariableName=delay_bram_din_lo_5  SampleTime=-1  SaveFormat=Structure With Time
  toWorkspace6 : ToWorkspace  VariableName=delay_bram_din_lo_6  SampleTime=-1  SaveFormat=Structure With Time
  toWorkspace7 : ToWorkspace  VariableName=delay_bram_din_lo_7  SampleTime=-1  SaveFormat=Structure With Time
  toWorkspace8 : ToWorkspace  VariableName=delay_bram_din_lo_8  SampleTime=-1  SaveFormat=Structure With Time
  toWorkspace9 : ToWorkspace  VariableName=delay_bram_din_lo_9  SampleTime=-1  SaveFormat=Structure With Time
  msb_out32 : Outport
  out31 : Outport  Port=2
  out30 : Outport  Port=3
  out29 : Outport  Port=4
  out28 : Outport  Port=5
  out27 : Outport  Port=6
  out26 : Outport  Port=7
  out25 : Outport  Port=8
  out24 : Outport  Port=9
  out23 : Outport  Port=10
  out22 : Outport  Port=11
  out21 : Outport  Port=12
  out20 : Outport  Port=13
  out19 : Outport  Port=14
  out18 : Outport  Port=15
  out17 : Outport  Port=16
  out16 : Outport  Port=17
  out15 : Outport  Port=18
  out14 : Outport  Port=19
  out13 : Outport  Port=20
  out12 : Outport  Port=21
  out11 : Outport  Port=22
  out10 : Outport  Port=23
  out9 : Outport  Port=24
  out8 : Outport  Port=25
  out7 : Outport  Port=26
  out6 : Outport  Port=27
  out5 : Outport  Port=28
  out4 : Outport  Port=29
  out3 : Outport  Port=30
  out2 : Outport  Port=31
  lsb_out1 : Outport  Port=32
  wires:
  bus_in/1 -> slice32/1, slice31/1, slice30/1, slice29/1, slice28/1, slice27/1, slice26/1, slice25/1, slice24/1, slice23/1, slice22/1, slice21/1, slice20/1, slice19/1, slice18/1, slice17/1, slice16/1, slice15/1, slice14/1, slice13/1, slice12/1, slice11/1, slice10/1, slice9/1, slice8/1, slice7/1, slice6/1, slice5/1, slice4/1, slice3/1, slice2/1, slice1/1
  slice32/1 -> reinterpret32/1
  reinterpret32/1 -> gatewayOut32/1, msb_out32/1
  gatewayOut32/1 -> toWorkspace32/1
  slice31/1 -> reinterpret31/1
  reinterpret31/1 -> gatewayOut31/1, out31/1
  gatewayOut31/1 -> toWorkspace31/1
  slice30/1 -> reinterpret30/1
  reinterpret30/1 -> gatewayOut30/1, out30/1
  gatewayOut30/1 -> toWorkspace30/1
  slice29/1 -> reinterpret29/1
  reinterpret29/1 -> gatewayOut29/1, out29/1
  gatewayOut29/1 -> toWorkspace29/1
  slice28/1 -> reinterpret28/1
  reinterpret28/1 -> gatewayOut28/1, out28/1
  gatewayOut28/1 -> toWorkspace28/1
  slice27/1 -> reinterpret27/1
  reinterpret27/1 -> gatewayOut27/1, out27/1
  gatewayOut27/1 -> toWorkspace27/1
  slice26/1 -> reinterpret26/1
  reinterpret26/1 -> gatewayOut26/1, out26/1
  gatewayOut26/1 -> toWorkspace26/1
  slice25/1 -> reinterpret25/1
  reinterpret25/1 -> gatewayOut25/1, out25/1
  gatewayOut25/1 -> toWorkspace25/1
  slice24/1 -> reinterpret24/1
  reinterpret24/1 -> gatewayOut24/1, out24/1
  gatewayOut24/1 -> toWorkspace24/1
  slice23/1 -> reinterpret23/1
  reinterpret23/1 -> gatewayOut23/1, out23/1
  gatewayOut23/1 -> toWorkspace23/1
  slice22/1 -> reinterpret22/1
  reinterpret22/1 -> gatewayOut22/1, out22/1
  gatewayOut22/1 -> toWorkspace22/1
  slice21/1 -> reinterpret21/1
  reinterpret21/1 -> gatewayOut21/1, out21/1
  gatewayOut21/1 -> toWorkspace21/1
  slice20/1 -> reinterpret20/1
  reinterpret20/1 -> gatewayOut20/1, out20/1
  gatewayOut20/1 -> toWorkspace20/1
  slice19/1 -> reinterpret19/1
  reinterpret19/1 -> gatewayOut19/1, out19/1
  gatewayOut19/1 -> toWorkspace19/1
  slice18/1 -> reinterpret18/1
  reinterpret18/1 -> gatewayOut18/1, out18/1
  gatewayOut18/1 -> toWorkspace18/1
  slice17/1 -> reinterpret17/1
  reinterpret17/1 -> gatewayOut17/1, out17/1
  gatewayOut17/1 -> toWorkspace17/1
  slice16/1 -> reinterpret16/1
  reinterpret16/1 -> gatewayOut16/1, out16/1
  gatewayOut16/1 -> toWorkspace16/1
  slice15/1 -> reinterpret15/1
  reinterpret15/1 -> gatewayOut15/1, out15/1
  gatewayOut15/1 -> toWorkspace15/1
  slice14/1 -> reinterpret14/1
  reinterpret14/1 -> gatewayOut14/1, out14/1
  gatewayOut14/1 -> toWorkspace14/1
  slice13/1 -> reinterpret13/1
  reinterpret13/1 -> gatewayOut13/1, out13/1
  gatewayOut13/1 -> toWorkspace13/1
  slice12/1 -> reinterpret12/1
  reinterpret12/1 -> gatewayOut12/1, out12/1
  gatewayOut12/1 -> toWorkspace12/1
  slice11/1 -> reinterpret11/1
  reinterpret11/1 -> gatewayOut11/1, out11/1
  gatewayOut11/1 -> toWorkspace11/1
  slice10/1 -> reinterpret10/1
  reinterpret10/1 -> gatewayOut10/1, out10/1
  gatewayOut10/1 -> toWorkspace10/1
  slice9/1 -> reinterpret9/1
  reinterpret9/1 -> gatewayOut9/1, out9/1
  gatewayOut9/1 -> toWorkspace9/1
  slice8/1 -> reinterpret8/1
  reinterpret8/1 -> gatewayOut8/1, out8/1
  gatewayOut8/1 -> toWorkspace8/1
  slice7/1 -> reinterpret7/1
  reinterpret7/1 -> gatewayOut7/1, out7/1
  gatewayOut7/1 -> toWorkspace7/1
  slice6/1 -> reinterpret6/1
  reinterpret6/1 -> gatewayOut6/1, out6/1
  gatewayOut6/1 -> toWorkspace6/1
  slice5/1 -> reinterpret5/1
  reinterpret5/1 -> gatewayOut5/1, out5/1
  gatewayOut5/1 -> toWorkspace5/1
  slice4/1 -> reinterpret4/1
  reinterpret4/1 -> gatewayOut4/1, out4/1
  gatewayOut4/1 -> toWorkspace4/1
  slice3/1 -> reinterpret3/1
  reinterpret3/1 -> gatewayOut3/1, out3/1
  gatewayOut3/1 -> toWorkspace3/1
  slice2/1 -> reinterpret2/1
  reinterpret2/1 -> gatewayOut2/1, out2/1
  gatewayOut2/1 -> toWorkspace2/1
  slice1/1 -> reinterpret1/1
  reinterpret1/1 -> gatewayOut1/1, lsb_out1/1
  gatewayOut1/1 -> toWorkspace1/1
